simulink model "Num1BD_reduced"  (R2023b)
settings: Solver=FixedStepAuto  StartTime=0.0  StopTime=10.0  RelTol=1e-3
settings Model: Creator=lyndo  LastModifiedBy=lyndo

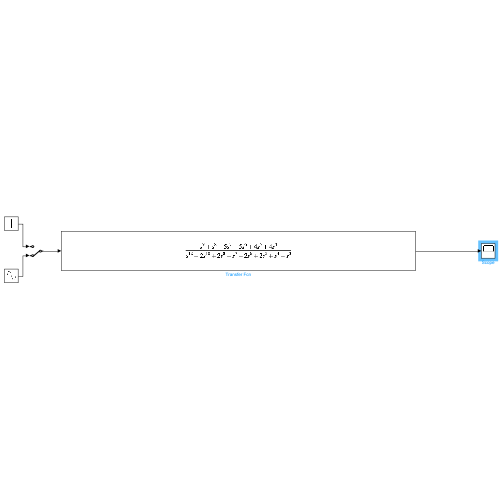
[thumbnail: Simulink's stored preview of the top-level diagram]
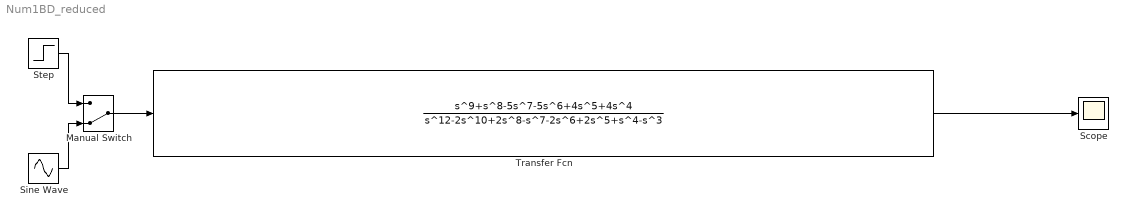
== system Num1BD_reduced ==
  Manual Switch : ManualSwitch  CurrentSetting=0
  Scope : Scope
  Sine Wave : Sin  SampleTime=0
  Step : Step  SampleTime=0
  Transfer Fcn : TransferFcn  Numerator="[0     0     0     1     1    -5    -5     4     4     0     0     0     0]"  Denominator="[1     0    -2     0     2    -1    -2     2     1    -1     0     0     0]"
  wires:
  Manual Switch/1 -> Transfer Fcn/1
  Step/1 -> Manual Switch/1
  Sine Wave/1 -> Manual Switch/2
  Transfer Fcn/1 -> Scope/1
